simulink model "exampleThermalNodeTHB"  (R2018b)
settings: Solver=ode45  StartTime=0.0  StopTime=3600  MaxStep=60  RelTol=1e-3  EnableMultiTasking=on
libraries: carnot x4, simulink x2
settings Model: Creator=drhf  LastModifiedBy=drhf
settings DataIOCC: LimitDataPoints=on  SaveFormat=Array  SignalLoggingSaveFormat=ModelDataLogs
settings OptimizationCC: ExpressionDepthLimit=2147483647  LifeSpan=inf
settings DebuggingCC: UnderspecifiedInitializationDetection=Classic  MergeDetectMultiDrivingBlocksExec=none  SolverPrmCheckMsg=warning  FcnCallInpInsideContextMsg=warning  StateNameClashWarn=warning  SFUnexpectedBacktrackingDiag=warning  SFNoUnconditionalDefaultTransitionDiag=warning  SFExecutionAtInitializationDiag=none
settings HardwareCC: ProdBitPerPointer=32  ProdBitPerSizeT=32  ProdBitPerPtrDiffT=32  ProdLargestAtomicFloat=None  ProdIntDivRoundTo=Undefined  ProdEndianess=Unspecified  ProdWordSize=32  ProdHWDeviceType=32-bit Generic
settings ModelReferenceCC: PropagateSignalLabelsOutOfModel=off
settings SFSimCC: SimUseLocalCustomCode=off
settings RTWCC: RTWUseLocalCustomCode=off
settings CodeAppCC: StateflowObjectComments=on
settings GRTTargetCC: TargetLangStandard=C89/C90 (ANSI)  GeneratePreprocessorConditionals=Disable all  CombineOutputUpdateFcns=off  GRTInterface=on
settings ConfigComp: CovMetricSettings=dw  CovHtmlReporting=on  CovSaveCumulativeToWorkspaceVar=on  CovSaveSingleToWorkspaceVar=on  CovExternalEMLEnable=off

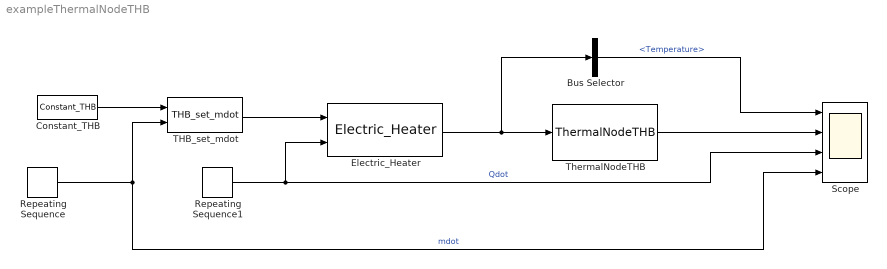
== system exampleThermalNodeTHB ==
  Bus Selector : BusSelector  OutputSignals=Temperature
  Constant_THB : carnot/Source/Simple/Constant_THB  t=20  mdot=0  p=1e5  mID=No Pressure Drop  fluid=Water  mix=0  mix2=0  mix3=0  dia=0.02  hgt=0
      settings: SourceProductName=Carnot
  Electric_Heater : carnot/Source/Boiler/Electric_Heater
      settings: SourceProductName=Carnot
  Repeating Sequence : simulink/Sources/Repeating Sequence  rep_seq_t=[0 900 901 3601]  rep_seq_y=[0 0 0.1 0.1]
  Repeating Sequence1 : simulink/Sources/Repeating Sequence  rep_seq_t=[0 2000 2001 3601]  rep_seq_y=[0 0 5000 5000]
  Scope : Scope  NumInputPorts=4
  THB_set_mdot : carnot/Source/Simple/THB_set_mdot
      settings: SourceProductName=Carnot
  ThermalNodeTHB : carnot/Basic/Thermal_Models/ThermalNodeTHB  UA=1  mcp=4182  Value=20
      settings: SourceProductName=Carnot
  wires:
  Repeating Sequence/1 -> THB_set_mdot/2, Scope/4  "mdot"
  Constant_THB/1 -> THB_set_mdot/1
  THB_set_mdot/1 -> Electric_Heater/1
  Electric_Heater/1 -> Bus Selector/1, ThermalNodeTHB/1
  ThermalNodeTHB/1 -> Scope/2
  Repeating Sequence1/1 -> Electric_Heater/2, Scope/3  "Qdot"
  Bus Selector/1 -> Scope/1  "<Temperature>"
